simulink model "sensors"  (R2023a)
settings: Solver=ode4  StartTime=0.0  StopTime=10.0  FixedStep=dt  RelTol=1e-3
undefined symbols (not defined in the file): dt, plant
settings Model: Creator=ndelurgio  LastModifiedBy=ndelurgio
settings DebuggingCC: ModelReferenceExtraNoncontSigs=none

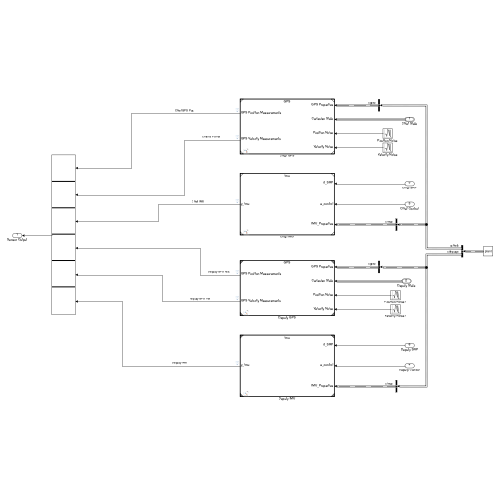
[thumbnail: Simulink's stored preview of the top-level diagram]
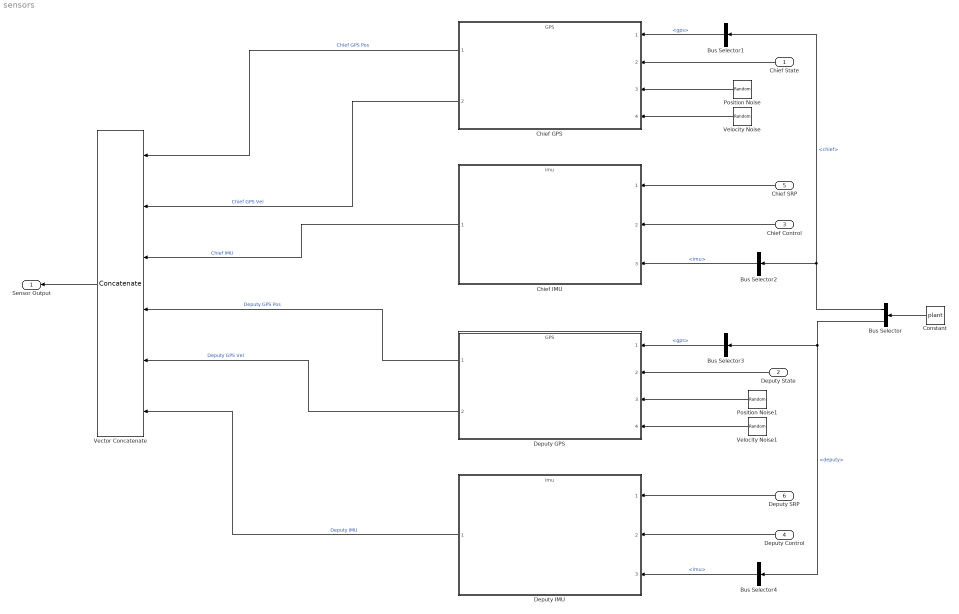
== system sensors ==
  Chief State : Inport  OutDataTypeStr=Bus: cartesianState
  Deputy State : Inport  Port=2  OutDataTypeStr=Bus: cartesianState
  Chief Control : Inport  Port=3  PortDimensions=3
  Deputy Control : Inport  Port=4  PortDimensions=3
  Chief SRP : Inport  Port=5  PortDimensions=3
  Deputy SRP : Inport  Port=6  PortDimensions=3
  Bus Selector : BusSelector  OutputSignals=chief,deputy
  Bus Selector1 : BusSelector  OutputSignals=properties.sensors.gps
  Bus Selector2 : BusSelector  OutputSignals=properties.sensors.imu
  Bus Selector3 : BusSelector  OutputSignals=properties.sensors.gps
  Bus Selector4 : BusSelector  OutputSignals=properties.sensors.imu
  Chief GPS : ModelReference  ModelNameDialog=GPS  SimulationMode=Normal  ModelReferenceVersion=1.20
  Chief IMU : ModelReference  ModelNameDialog=imu  SimulationMode=Normal  ModelReferenceVersion=1.19
  Constant : Constant  Value=plant  OutDataTypeStr=Bus: plantBus
  Deputy GPS : ModelReference  ModelNameDialog=GPS  SimulationMode=Normal  ModelReferenceVersion=1.20
  Deputy IMU : ModelReference  ModelNameDialog=imu  SimulationMode=Normal  ModelReferenceVersion=1.19
  Position Noise : RandomNumber  Mean=[0;0;0]  Variance=[1;1;1]  Seed=[5;3;22]  SampleTime=dt
  Position Noise1 : RandomNumber  Mean=[0;0;0]  Variance=[1;1;1]  Seed=[5;3;22]  SampleTime=dt
  Vector Concatenate : Concatenate  NumInputs=6
  Velocity Noise : RandomNumber  Mean=[0;0;0]  Variance=[1;1;1]  Seed=[2;8;14]  SampleTime=dt
  Velocity Noise1 : RandomNumber  Mean=[0;0;0]  Variance=[1;1;1]  Seed=[2;8;14]  SampleTime=dt
  Sensor Output : Outport
  wires:
  Constant/1 -> Bus Selector/1
  Bus Selector/1 -> Bus Selector1/1, Bus Selector2/1  "<chief>"
  Bus Selector1/1 -> Chief GPS/1  "<gps>"
  Chief State/1 -> Chief GPS/2
  Chief SRP/1 -> Chief IMU/1
  Chief Control/1 -> Chief IMU/2
  Bus Selector2/1 -> Chief IMU/3  "<imu>"
  Bus Selector3/1 -> Deputy GPS/1  "<gps>"
  Bus Selector/2 -> Bus Selector4/1, Bus Selector3/1  "<deputy>"
  Deputy State/1 -> Deputy GPS/2
  Deputy SRP/1 -> Deputy IMU/1
  Deputy Control/1 -> Deputy IMU/2
  Bus Selector4/1 -> Deputy IMU/3  "<imu>"
  Chief GPS/1 -> Vector Concatenate/1  "Chief GPS Pos"
  Chief GPS/2 -> Vector Concatenate/2  "Chief GPS Vel"
  Deputy GPS/1 -> Vector Concatenate/4  "Deputy GPS Pos"
  Deputy GPS/2 -> Vector Concatenate/5  "Deputy GPS Vel"
  Deputy IMU/1 -> Vector Concatenate/6  "Deputy IMU"
  Chief IMU/1 -> Vector Concatenate/3  "Chief IMU"
  Vector Concatenate/1 -> Sensor Output/1
  Position Noise/1 -> Chief GPS/3
  Velocity Noise/1 -> Chief GPS/4
  Velocity Noise1/1 -> Deputy GPS/4
  Position Noise1/1 -> Deputy GPS/3
